simulink model "nivel1"  (R2018b)
settings: Solver=VariableStepAuto  StartTime=0.0  StopTime=10.0  RelTol=1e-3
libraries: fuzblock x1
settings Model: Creator=seba  LastModifiedBy=seba

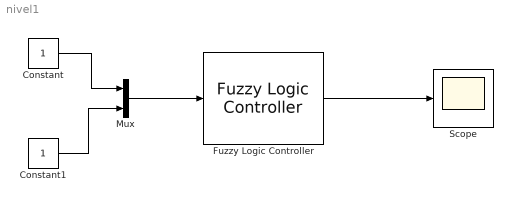
== system nivel1 ==
  Constant : Constant
  Constant1 : Constant
  Fuzzy Logic Controller : fuzblock/Fuzzy Logic  Controller  FIS=nivel1  OutputSampleNumber=101  DataType=double  FuzzifiedInputs=off  RuleFiringStrengths=off  RuleOutputs=off  AggregatedOutputs=off  SimulateUsing=Interpreted execution  OutOfRangeInputValueMessage=warning  NoRuleFiredMessage=warning  EmptyOutputFuzzySetMessage=warning
  Mux : Mux  Inputs=2
  Scope : Scope
  wires:
  Mux/1 -> Fuzzy Logic Controller/1
  Fuzzy Logic Controller/1 -> Scope/1
  Constant/1 -> Mux/1
  Constant1/1 -> Mux/2
